simulink model "kls_motor_test_host"  (R2025b)
settings: Solver=FixedStepAuto  StartTime=0.0  StopTime=inf  FixedStep=0.001  RelTol=1e-3
libraries: instrumentseriallib x3, svdutilitieslib x1
settings Model: Creator=erik  LastModifiedBy=orang

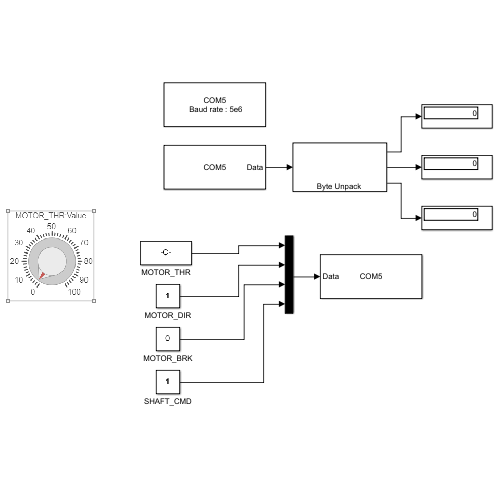
[thumbnail: Simulink's stored preview of the top-level diagram]
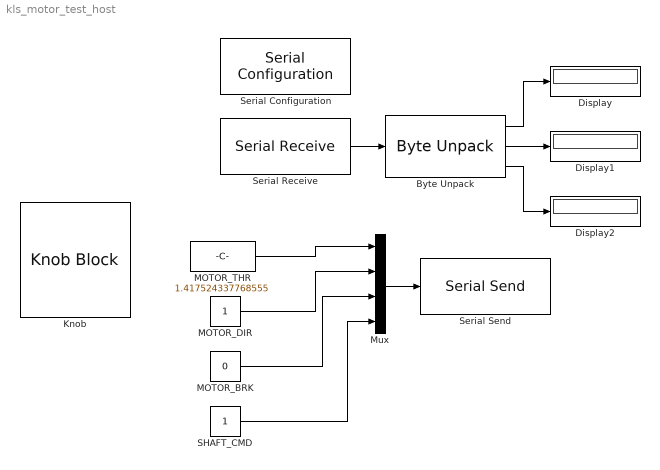
== system kls_motor_test_host ==
  Byte Unpack : svdutilitieslib/Byte Unpack  dimensions={[1],[1],[1]}  datatypes={'uint16' 'uint16' 'uint8'}  byteAlign=1  blockPlatform=tic2000
      settings: LibrarySourceBlock=c2000lib/Target Communication/Byte Unpack
  Display : Display
  Display1 : Display
  Display2 : Display
  Knob : KnobBlock  TickInterval=10
  MOTOR_BRK : Constant  Value=0  OutDataTypeStr=uint8
  MOTOR_DIR : Constant  OutDataTypeStr=uint8
  MOTOR_THR : Constant  Value=1.417524337768555  OutDataTypeStr=uint8  SampleTime=0.1
  Mux : Mux
  "SHAFT_CMD " : Constant  OutDataTypeStr=uint8
  Serial Configuration : instrumentseriallib/Serial Configuration  Priority=-200000  PortSel=COM5  Port=COM5  ComPort=COM5  BaudRate=5e6  DataBits=8  Parity=none  StopBits=1  ByteOrder=little-endian  FlowControl=none  Timeout=10  SimulateUsing=Interpreted execution  BlockInModel=on  aMode=1
      settings: LibrarySourceBlock=c2000lib/Host Communication/Serial Configuration
  Serial Receive : instrumentseriallib/Serial Receive  Priority=1  PortSel=COM5  Port=COM5  ComPort=COM5  DataType=uint8  SaveDataType=uint8  ToggleHeader=off  Header=[]  ToggleDataSize=on  DataSize=[5 1]  ToggleTerminator=off  Terminator=<none>  CustomTerminator=[]  InputFormat=Column major  EnableBlockingMode=on  ActionDataUnavailable=Error  ActionWhenDataUnavailable=Error  CustomValue=0  SampleTime=0.001  SimulateUsing=Interpreted execution  BlockInModel=on  aMode=1  LibraryInUse=c2000lib
      settings: LibrarySourceBlock=c2000lib/Host Communication/Serial Receive
  Serial Send : instrumentseriallib/Serial Send  Priority=1  PortSel=COM5  Port=COM5  ComPort=COM5  Header=[]  Terminator=<none>  CustomTerminator=[]  EnableBlockingMode=off  SimulateUsing=Interpreted execution  BlockInModel=on  aMode=1
      settings: LibrarySourceBlock=c2000lib/Host Communication/Serial Send
  wires:
  MOTOR_THR/1 -> Mux/1
  MOTOR_DIR/1 -> Mux/2
  MOTOR_BRK/1 -> Mux/3
  "SHAFT_CMD "/1 -> Mux/4
  Mux/1 -> Serial Send/1
  Serial Receive/1 -> Byte Unpack/1
  Byte Unpack/1 -> Display/1
  Byte Unpack/2 -> Display1/1
  Byte Unpack/3 -> Display2/1
